simulink model "Pcontrol"  (R2019a)
settings: Solver=VariableStepAuto  StartTime=0.0  StopTime=10.0  MaxStep=1e-3  RelTol=1e-3
values from neighbouring files (symbols this model uses):
  K = 100    [cruiseControlExample.m]
  r = 100*ones(size(t))    [cruiseControlExample.m]
settings Model: Creator=adria  LastModifiedBy=adria

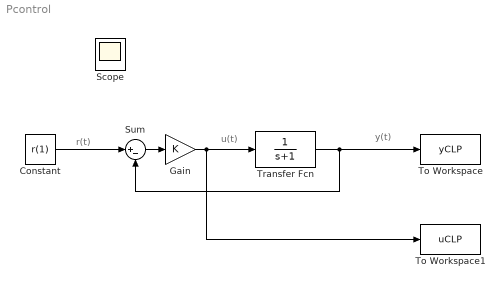
== system Pcontrol ==
  note: r(t)
  note: y(t)
  note: u(t)
  Constant : Constant  Value=r(1)
  Gain : Gain  Gain=K
  Sum : Sum  Inputs=|+-
  To Workspace : ToWorkspace  VariableName=yCLP  SaveFormat=Structure With Time  SampleTime=-1
  To Workspace1 : ToWorkspace  VariableName=uCLP  SaveFormat=Structure With Time  SampleTime=-1
  Transfer Fcn : TransferFcn  Denominator=[1 1]
  Scope : Scope
  wires:
  Gain/1 -> To Workspace1/1, Transfer Fcn/1
  Sum/1 -> Gain/1
  Constant/1 -> Sum/1
  Transfer Fcn/1 -> To Workspace/1, Sum/2
